simulink model "UVLamp"  (R2020a)
settings: Solver=VariableStepAuto  StartTime=0.0  StopTime=10.0  RelTol=1e-3
libraries: powerlib x18, powerlib_meascontrol x2
settings Model: Creator=susha  LastModifiedBy=susha

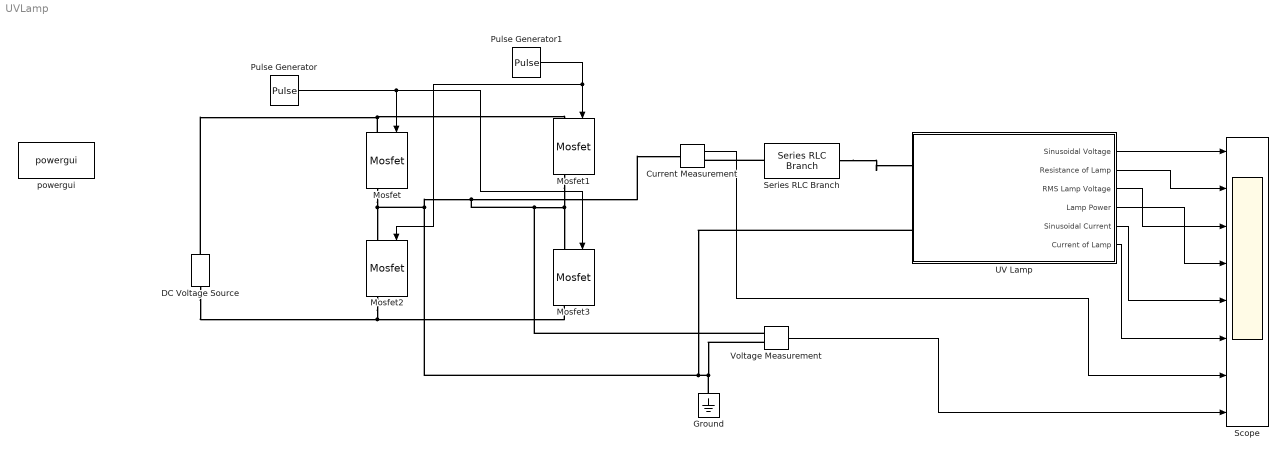
== system UVLamp ==
  Current Measurement : powerlib/Measurements/Current Measurement  PhasorSimulation=off  OutputType=Complex  PSBequivalent=0
  DC Voltage Source : powerlib/Electrical Sources/DC Voltage Source  Amplitude=200  Measurements=None
  Ground : powerlib/Elements/Ground  LConnTagsString=a
  Mosfet{,1..3} (4 alike) : powerlib/Power Electronics/Mosfet  Ron=0.1  Lon=0  Rd=0.01  Vfd=0  IC=0  Rs=1e5  Cs=inf  Measurements=on
  Pulse Generator : DiscretePulseGenerator  PulseType=Time based  Period=2e-3  PulseWidth=50
  Pulse Generator1 : DiscretePulseGenerator  PulseType=Time based  Period=2e-3  PulseWidth=50  PhaseDelay=1e-3
  Scope : Scope  NumInputPorts=8
  Series RLC Branch : powerlib/Elements/Series RLC Branch  LConnTagsString=__new0  RConnTagsString=__new0  BranchType=LC  Resistance=0  Inductance=1.31e-3  SetiL0=off  InitialCurrent=0  Capacitance=14.4e-9  Setx0=off  InitialVoltage=0  Measurements=None
  UV Lamp : Subsystem
  Voltage Measurement : powerlib/Measurements/Voltage Measurement  PhasorSimulation=off  OutputType=Complex  PSBequivalent=0
  powergui : powerlib/powergui  Priority=1  SimulationMode=Continuous  SampleTime=50e-6  frequency=60  Iterations=50  frequencyindice=0  Pbase=100e6  ErrMax=1e-4  UnitsV=kV  UnitsW=MW  buscounter=0  FunctionMessages=off  echomessages=off  EnableUseOfTLC=off  CurrentSourceSwitches=off  DisableSnubberDevices=off  DisableRonSwitches=off  DisableVfSwitches=off  DisplayEquations=off  AutomaticDiscreteSolvers=off  SolverType=Tustin/Backward Euler (TBE)  Interpol=off  ExternalGateDelay=off  methode=off  Ts=100  x0status=blocks  SPID=on  SwTol=0  HookPort=off  NonlinearTolerance=1e-4  nMaxIteration=100  ContinueOnMaxIteration=off  RestoreLinks=warning  ResistiveCurrentMeasurement=off  Frange=[0:2:500]  Ylog=off  Xlog=on  ShowGrid=off  save=off  variable=ZData  structure=0  ZoomFFT=off  StartTime=0.0  cycles=1  DisplayStyle=1  fundamental=60  FreqAxis=off  MaxFrequency=1000  frequencyindicesteady=1  RmsSteady=1  display=off
  wires:
  Pulse Generator/1 -> Mosfet/1, Mosfet3/1
  Pulse Generator1/1 -> Mosfet2/1, Mosfet1/1
  UV Lamp/1(Sinusoidal Voltage) -> Scope/1
  UV Lamp/2(Resistance of Lamp) -> Scope/2
  UV Lamp/3(RMS Lamp Voltage) -> Scope/3
  UV Lamp/4(Lamp Power) -> Scope/4
  UV Lamp/5(Sinusoidal Current) -> Scope/5
  UV Lamp/6(Current of Lamp) -> Scope/6
  Current Measurement/1 -> Scope/7
  Voltage Measurement/1 -> Scope/8
  connections:
  Mosfet1/RConn1 -- Current Measurement/LConn1 -- Ground/LConn1 -- Voltage Measurement/LConn2 -- UV Lamp/LConn2 -- Mosfet2/LConn1 -- Mosfet/RConn1 -- Voltage Measurement/LConn1 -- Mosfet3/LConn1
  Mosfet/LConn1 -- DC Voltage Source/RConn1 -- Mosfet1/LConn1
  Mosfet2/RConn1 -- DC Voltage Source/LConn1 -- Mosfet3/RConn1
  Series RLC Branch/LConn1 -- Current Measurement/RConn1
  Series RLC Branch/RConn1 -- UV Lamp/LConn1

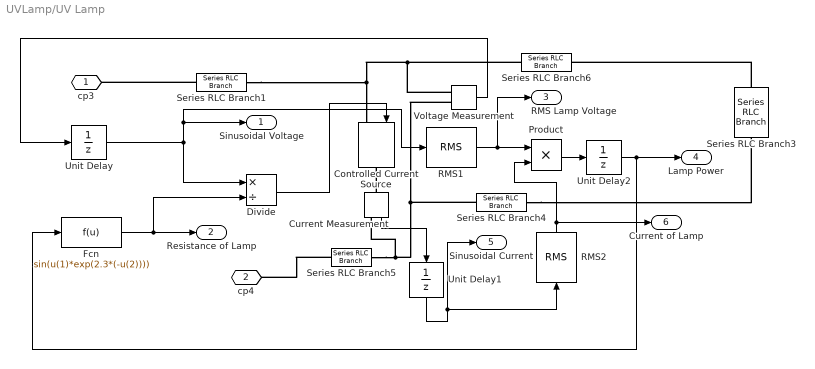
== system UVLamp/UV Lamp ==
  Controlled Current Source : powerlib/Electrical Sources/Controlled Current Source  Initialize=on  Source_Type=AC  Amplitude=0  Phase=0  Frequency=0  Measurements=None
  Current Measurement : powerlib/Measurements/Current Measurement  PhasorSimulation=off  OutputType=Complex  PSBequivalent=0
  Divide : Product  Inputs=*/
  Fcn : Fcn  Expr=sin(u(1)*exp(2.3*(-u(2))))
  Product : Product
  RMS1 : powerlib_meascontrol/Measurements/RMS  TrueRMS=on  Freq=60  RMSInit=120  Ts=0
  RMS2 : powerlib_meascontrol/Measurements/RMS  TrueRMS=on  Freq=60  RMSInit=120  Ts=0
  Series RLC Branch{1,4..6} (4 alike) : powerlib/Elements/Series RLC Branch  LConnTagsString=__new0  RConnTagsString=__new0  BranchType=R  Resistance=6  Inductance=1.31e-3  SetiL0=off  InitialCurrent=0  Capacitance=14.4e-9  Setx0=off  InitialVoltage=0  Measurements=None
  Series RLC Branch3 : powerlib/Elements/Series RLC Branch  LConnTagsString=__new0  RConnTagsString=__new0  BranchType=C  Resistance=6  Inductance=1.31e-3  SetiL0=off  InitialCurrent=0  Capacitance=2.97e-9  Setx0=off  InitialVoltage=0  Measurements=None
  Unit Delay : UnitDelay  SampleTime=-1  HasFrameUpgradeWarning=on
  Unit Delay1 : UnitDelay  SampleTime=-1  HasFrameUpgradeWarning=on
  Unit Delay2 : UnitDelay  SampleTime=-1  HasFrameUpgradeWarning=on
  Voltage Measurement : powerlib/Measurements/Voltage Measurement  PhasorSimulation=off  OutputType=Complex  PSBequivalent=0
  cp3 : PMIOPort  Side=Left
  cp4 : PMIOPort  Port=2  Side=Left
  Sinusoidal Voltage : Outport
  Resistance of Lamp : Outport  Port=2
  RMS Lamp Voltage : Outport  Port=3
  Lamp Power : Outport  Port=4
  Sinusoidal Current : Outport  Port=5
  Current of Lamp : Outport  Port=6
  wires:
  Unit Delay/1 -> RMS1/1, Sinusoidal Voltage/1, Divide/1
  Fcn/1 -> Divide/2, Resistance of Lamp/1
  Current Measurement/1 -> Unit Delay1/1
  Divide/1 -> Controlled Current Source/1
  RMS1/1 -> RMS Lamp Voltage/1, Product/1
  Product/1 -> Unit Delay2/1
  Unit Delay2/1 -> Fcn/1, Lamp Power/1
  Unit Delay1/1 -> RMS2/1, Sinusoidal Current/1
  RMS2/1 -> Product/2, Current of Lamp/1
  Voltage Measurement/1 -> Unit Delay/1
  connections:
  Series RLC Branch1/RConn1 -- Voltage Measurement/LConn1 -- Series RLC Branch6/LConn1 -- Controlled Current Source/LConn1
  Series RLC Branch1/LConn1 -- cp3/RConn1
  Series RLC Branch5/LConn1 -- cp4/RConn1
  Series RLC Branch5/RConn1 -- Series RLC Branch4/LConn1 -- Voltage Measurement/LConn2 -- Current Measurement/RConn1
  Current Measurement/LConn1 -- Controlled Current Source/RConn1
  Series RLC Branch3/LConn1 -- Series RLC Branch6/RConn1
  Series RLC Branch4/RConn1 -- Series RLC Branch3/RConn1
